simulink model "Task_1_c"  (R2024b)
settings: Solver=ode4  StartTime=0.0  StopTime=1000.0  FixedStep=0.01  RelTol=1e-3
settings Model: Creator=max  LastModifiedBy=max

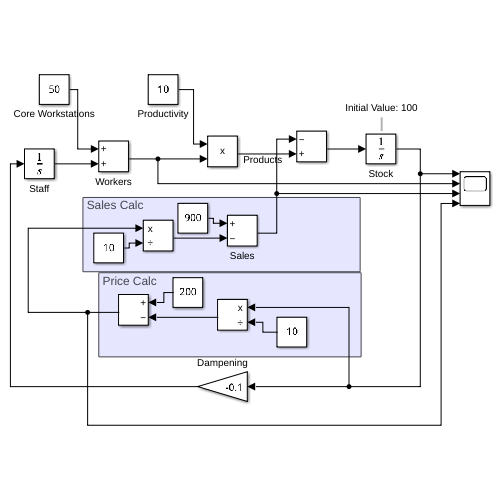
[thumbnail: Simulink's stored preview of the top-level diagram]
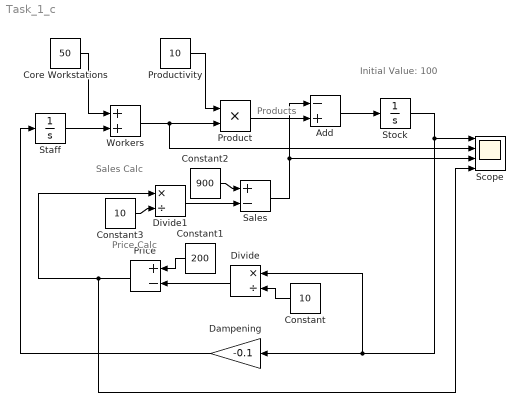
== system Task_1_c ==
  note: Sales Calc
  note: Price Calc
  note: Products
  note: Initial Value: 100
  Add : Sum  Inputs=-+
  Constant : Constant  Value=10
  Constant1 : Constant  Value=200
  Constant2 : Constant  Value=900
  Constant3 : Constant  Value=10
  Core Workstations : Constant  Value=50
  Dampening : Gain  Gain=-0.1
  Divide : Product  Inputs=*/
  Divide1 : Product  Inputs=*/
  Price : Sum  Inputs=+-
  Product : Product
  Productivity : Constant  Value=10
  Sales : Sum  Inputs=+-
  Scope : Scope  NumInputPorts=4
  Staff : Integrator
  Stock : Integrator  InitialCondition=100
  Workers : Sum
  wires:
  Add/1 -> Stock/1
  Product/1 -> Add/2
  Productivity/1 -> Product/1
  Stock/1 -> Divide/1, Dampening/1, Scope/1
  Dampening/1 -> Staff/1
  Staff/1 -> Workers/2
  Workers/1 -> Scope/2, Product/2
  Core Workstations/1 -> Workers/1
  Constant/1 -> Divide/2
  Divide/1 -> Price/2
  Constant1/1 -> Price/1
  Price/1 -> Scope/4, Divide1/1
  Constant3/1 -> Divide1/2
  Divide1/1 -> Sales/2
  Constant2/1 -> Sales/1
  Sales/1 -> Add/1, Scope/3
